simulink model "P702_NI_SoftECU"  (R2019a)
settings: Solver=ode1  StartTime=0.0  StopTime=Inf  FixedStep=0.001  RelTol=1e-3  EnableMultiTasking=on
PreLoadFcn:
  | run '.\VeriStand_BlockSet\NIVeriStandAddPaths.m'
undefined symbols (not defined in the file or in its folder): magnitude
libraries: simulink x83, simulink_extras x1
(part 64 of 76)

== system P702_NI_SoftECU/Output/Subsystem1/CAN_Signal/ABS_ESC/Global_PATS_SubTarget_0x49 ==
  in_port : Inport
  bus_selector : BusSelector  OutputSignals=immoSubTarget1Cmd_T1,immoSubTarget1Data_T1
  immoSubTarget1Cmd_T1 : Terminator
  immoSubTarget1Data_T1 : Terminator
  wires:
  in_port/1 -> bus_selector/1  "Subsystem1"
  bus_selector/1 -> immoSubTarget1Cmd_T1/1  "<immoSubTarget1Cmd_T1>"
  bus_selector/2 -> immoSubTarget1Data_T1/1  "<immoSubTarget1Data_T1>"

== system P702_NI_SoftECU/Output/Subsystem1/CAN_Signal/ABS_ESC/SelectDriveModeData2_0x44E ==
  in_port : Inport
  SelDrvMdePos01_D_Stat : Terminator
  SelDrvMdePos02_D_Stat : Terminator
  SelDrvMdePos03_D_Stat : Terminator
  SelDrvMdePos04_D_Stat : Terminator
  SelDrvMdePos05_D_Stat : Terminator
  SelDrvMdePos06_D_Stat : Terminator
  SelDrvMdePos07_D_Stat : Terminator
  SelDrvMdePos08_D_Stat : Terminator
  SelDrvMdePos09_D_Stat : Terminator
  SelDrvMdePos10_D_Stat : Terminator
  SelDrvMdePos11_D_Stat : Terminator
  SelDrvMdePos12_D_Stat : Terminator
  bus_selector : BusSelector  OutputSignals=SelDrvMdePos01_D_Stat,SelDrvMdePos02_D_Stat,SelDrvMdePos03_D_Stat,SelDrvMdePos04_D_Stat,SelDrvMdePos05_D_Stat,SelDrvMdePos06_D_Stat,SelDrvMdePos07_D_Stat,SelDrvMdePos12_D_Stat,SelDrvMdePos11_D_Stat,SelDrvMdePos10_D_Stat,SelDrvMdePos09_D_Stat,SelDrvMdePos08_D_Stat
  wires:
  in_port/1 -> bus_selector/1  "Subsystem1"
  bus_selector/1 -> SelDrvMdePos01_D_Stat/1  "<SelDrvMdePos01_D_Stat>"
  bus_selector/2 -> SelDrvMdePos02_D_Stat/1  "<SelDrvMdePos02_D_Stat>"
  bus_selector/3 -> SelDrvMdePos03_D_Stat/1  "<SelDrvMdePos03_D_Stat>"
  bus_selector/4 -> SelDrvMdePos04_D_Stat/1  "<SelDrvMdePos04_D_Stat>"
  bus_selector/5 -> SelDrvMdePos05_D_Stat/1  "<SelDrvMdePos05_D_Stat>"
  bus_selector/6 -> SelDrvMdePos06_D_Stat/1  "<SelDrvMdePos06_D_Stat>"
  bus_selector/7 -> SelDrvMdePos07_D_Stat/1  "<SelDrvMdePos07_D_Stat>"
  bus_selector/8 -> SelDrvMdePos12_D_Stat/1  "<SelDrvMdePos12_D_Stat>"
  bus_selector/9 -> SelDrvMdePos11_D_Stat/1  "<SelDrvMdePos11_D_Stat>"
  bus_selector/10 -> SelDrvMdePos10_D_Stat/1  "<SelDrvMdePos10_D_Stat>"
  bus_selector/11 -> SelDrvMdePos09_D_Stat/1  "<SelDrvMdePos09_D_Stat>"
  bus_selector/12 -> SelDrvMdePos08_D_Stat/1  "<SelDrvMdePos08_D_Stat>"

== system P702_NI_SoftECU/Output/Subsystem1/CAN_Signal/ABS_ESC/SelectDriveModeData_0x420 ==
  in_port : Inport
  ActvDrvMde_D2_Stat : Terminator
  AwdMde_D_RqBrk : Terminator
  SelDrvMdeMsgTxt_D_Rq : Terminator
  SelDrvMdePos01_B_Avail : Terminator
  SelDrvMdePos02_B_Avail : Terminator
  SelDrvMdePos03_B_Avail : Terminator
  SelDrvMdePos04_B_Avail : Terminator
  SelDrvMdePos05_B_Avail : Terminator
  SelDrvMdePos06_B_Avail : Terminator
  SelDrvMdePos07_B_Avail : Terminator
  SelDrvMdePos08_B_Avail : Terminator
  SelDrvMdePos09_B_Avail : Terminator
  SelDrvMdePos10_B_Avail : Terminator
  SelDrvMdePos11_B_Avail : Terminator
  SelDrvMdePos12_B_Avail : Terminator
  SelDrvMdePt_D_Rq : Terminator
  SelDrvMde_D2_Rq : Terminator
  SelDrvMde_D_Stat : Terminator
  bus_selector : BusSelector  OutputSignals=SelDrvMdeMsgTxt_D_Rq,SelDrvMdePt_D_Rq,SelDrvMde_D_Stat,SelDrvMdePos01_B_Avail,AwdMde_D_RqBrk,SelDrvMdePos02_B_Avail,SelDrvMdePos03_B_Avail,SelDrvMdePos04_B_Avail,SelDrvMdePos05_B_Avail,SelDrvMdePos06_B_Avail,SelDrvMdePos07_B_Avail,SelDrvMdePos08_B_Avail,SelDrvMdePos09_B_Avail,SelDrvMdePos10_B_Avail,SelDrvMdePos11_B_Avail,SelDrvMdePos12_B_Avail,ActvDrvMde_D2_Stat,SelDrvMde_D2_Rq
  wires:
  in_port/1 -> bus_selector/1  "Subsystem1"
  bus_selector/1 -> SelDrvMdeMsgTxt_D_Rq/1  "<SelDrvMdeMsgTxt_D_Rq>"
  bus_selector/2 -> SelDrvMdePt_D_Rq/1  "<SelDrvMdePt_D_Rq>"
  bus_selector/3 -> SelDrvMde_D_Stat/1  "<SelDrvMde_D_Stat>"
  bus_selector/4 -> SelDrvMdePos01_B_Avail/1  "<SelDrvMdePos01_B_Avail>"
  bus_selector/5 -> AwdMde_D_RqBrk/1  "<AwdMde_D_RqBrk>"
  bus_selector/6 -> SelDrvMdePos02_B_Avail/1  "<SelDrvMdePos02_B_Avail>"
  bus_selector/7 -> SelDrvMdePos03_B_Avail/1  "<SelDrvMdePos03_B_Avail>"
  bus_selector/8 -> SelDrvMdePos04_B_Avail/1  "<SelDrvMdePos04_B_Avail>"
  bus_selector/9 -> SelDrvMdePos05_B_Avail/1  "<SelDrvMdePos05_B_Avail>"
  bus_selector/10 -> SelDrvMdePos06_B_Avail/1  "<SelDrvMdePos06_B_Avail>"
  bus_selector/11 -> SelDrvMdePos07_B_Avail/1  "<SelDrvMdePos07_B_Avail>"
  bus_selector/12 -> SelDrvMdePos08_B_Avail/1  "<SelDrvMdePos08_B_Avail>"
  bus_selector/13 -> SelDrvMdePos09_B_Avail/1  "<SelDrvMdePos09_B_Avail>"
  bus_selector/14 -> SelDrvMdePos10_B_Avail/1  "<SelDrvMdePos10_B_Avail>"
  bus_selector/15 -> SelDrvMdePos11_B_Avail/1  "<SelDrvMdePos11_B_Avail>"
  bus_selector/16 -> SelDrvMdePos12_B_Avail/1  "<SelDrvMdePos12_B_Avail>"
  bus_selector/17 -> ActvDrvMde_D2_Stat/1  "<ActvDrvMde_D2_Stat>"
  bus_selector/18 -> SelDrvMde_D2_Rq/1  "<SelDrvMde_D2_Rq>"

== system P702_NI_SoftECU/Output/Subsystem1/CAN_Signal/ABS_ESC/SteeringPinion_Data2_0x7F ==
  in_port : Inport
  AwdLatDelta_B_Rq : Terminator
  AwdLatDelta_Tq_Rq : Terminator
  bus_selector : BusSelector  OutputSignals=AwdLatDelta_B_Rq,AwdLatDelta_Tq_Rq
  wires:
  in_port/1 -> bus_selector/1  "Subsystem1"
  bus_selector/1 -> AwdLatDelta_B_Rq/1  "<AwdLatDelta_B_Rq>"
  bus_selector/2 -> AwdLatDelta_Tq_Rq/1  "<AwdLatDelta_Tq_Rq>"

== system P702_NI_SoftECU/Output/Subsystem1/CAN_Signal/ABS_ESC/TesterPhysicalResABS_0x768 ==
  in_port : Inport
  TesterPhysicalResABS : Terminator
  bus_selector : BusSelector  OutputSignals=TesterPhysicalResABS
  wires:
  in_port/1 -> bus_selector/1  "Subsystem1"
  bus_selector/1 -> TesterPhysicalResABS/1  "<TesterPhysicalResABS>"

== system P702_NI_SoftECU/Output/Subsystem1/CAN_Signal/ABS_ESC/TrailerBrakeData_0x412 ==
  in_port : Inport
  TrlrBrk_Pc_Rq : Terminator
  VehPtch_An_Dsply : Terminator
  VehRol_An_Dsply : Terminator
  bus_selector : BusSelector  OutputSignals=TrlrBrk_Pc_Rq,VehPtch_An_Dsply,VehRol_An_Dsply
  wires:
  in_port/1 -> bus_selector/1  "Subsystem1"
  bus_selector/1 -> TrlrBrk_Pc_Rq/1  "<TrlrBrk_Pc_Rq>"
  bus_selector/2 -> VehPtch_An_Dsply/1  "<VehPtch_An_Dsply>"
  bus_selector/3 -> VehRol_An_Dsply/1  "<VehRol_An_Dsply>"

== system P702_NI_SoftECU/Output/Subsystem1/CAN_Signal/ABS_ESC/WheelData_0x216 ==
  in_port : Inport
  BrkObdData_No_Actl : Terminator
  BrkObdIndex_No_Actl : Terminator
  WhlDirFl_D_Actl : Terminator
  WhlDirFr_D_Actl : Terminator
  WhlDirRl_D_Actl : Terminator
  WhlDirRr_D_Actl : Terminator
  WhlRotatFl_No_Cnt : Terminator
  WhlRotatFr_No_Cnt : Terminator
  WhlRotatRl_No_Cnt : Terminator
  WhlRotatRr_No_Cnt : Terminator
  bus_selector : BusSelector  OutputSignals=WhlRotatFr_No_Cnt,WhlRotatFl_No_Cnt,WhlRotatRr_No_Cnt,WhlRotatRl_No_Cnt,WhlDirRl_D_Actl,WhlDirFr_D_Actl,WhlDirFl_D_Actl,WhlDirRr_D_Actl,BrkObdIndex_No_Actl,BrkObdData_No_Actl
  wires:
  in_port/1 -> bus_selector/1  "Subsystem1"
  bus_selector/1 -> WhlRotatFr_No_Cnt/1  "<WhlRotatFr_No_Cnt>"
  bus_selector/2 -> WhlRotatFl_No_Cnt/1  "<WhlRotatFl_No_Cnt>"
  bus_selector/3 -> WhlRotatRr_No_Cnt/1  "<WhlRotatRr_No_Cnt>"
  bus_selector/4 -> WhlRotatRl_No_Cnt/1  "<WhlRotatRl_No_Cnt>"
  bus_selector/5 -> WhlDirRl_D_Actl/1  "<WhlDirRl_D_Actl>"
  bus_selector/6 -> WhlDirFr_D_Actl/1  "<WhlDirFr_D_Actl>"
  bus_selector/7 -> WhlDirFl_D_Actl/1  "<WhlDirFl_D_Actl>"
  bus_selector/8 -> WhlDirRr_D_Actl/1  "<WhlDirRr_D_Actl>"
  bus_selector/9 -> BrkObdIndex_No_Actl/1  "<BrkObdIndex_No_Actl>"
  bus_selector/10 -> BrkObdData_No_Actl/1  "<BrkObdData_No_Actl>"

== system P702_NI_SoftECU/Output/Subsystem1/CAN_Signal/ABS_ESC/WheelSpeed_0x217 ==
  in_port : Inport
  WhlFl_W_Meas : Terminator
  WhlFr_W_Meas : Terminator
  WhlRl_W_Meas : Terminator
  WhlRr_W_Meas : Terminator
  bus_selector : BusSelector  OutputSignals=WhlFl_W_Meas,WhlFr_W_Meas,WhlRl_W_Meas,WhlRr_W_Meas
  wires:
  in_port/1 -> bus_selector/1  "Subsystem1"
  bus_selector/1 -> WhlFl_W_Meas/1  "<WhlFl_W_Meas>"
  bus_selector/2 -> WhlFr_W_Meas/1  "<WhlFr_W_Meas>"
  bus_selector/3 -> WhlRl_W_Meas/1  "<WhlRl_W_Meas>"
  bus_selector/4 -> WhlRr_W_Meas/1  "<WhlRr_W_Meas>"

== system P702_NI_SoftECU/Output/Subsystem1/CAN_Signal/ADAS/ACCDATA ==
  in_port : Inport
  AccBrkDecel_B_Rq : Terminator
  AccBrkPrchg_B_Rq : Terminator
  AccBrkTot_A_Rq : Terminator
  AccCancl_B_Rq : Terminator
  AccPrpl_A_Rq : Terminator
  AccPrpl_A_Rq1 : Terminator
  AccStopStat_B_Rq : Terminator
  CmbbEngTqMn_B_Rq : Terminator
  bus_selector : BusSelector  OutputSignals=AccBrkPrchg_B_Rq,AccBrkDecel_B_Rq,AccStopStat_B_Rq,AccBrkTot_A_Rq,CmbbEngTqMn_B_Rq,AccCancl_B_Rq,AccPrpl_A_Rq,AccPrpl_A_Rq1
  wires:
  in_port/1 -> bus_selector/1  "Subsystem1"
  bus_selector/1 -> AccBrkPrchg_B_Rq/1  "<AccBrkPrchg_B_Rq>"
  bus_selector/2 -> AccBrkDecel_B_Rq/1  "<AccBrkDecel_B_Rq>"
  bus_selector/3 -> AccStopStat_B_Rq/1  "<AccStopStat_B_Rq>"
  bus_selector/4 -> AccBrkTot_A_Rq/1  "<AccBrkTot_A_Rq>"
  bus_selector/5 -> CmbbEngTqMn_B_Rq/1  "<CmbbEngTqMn_B_Rq>"
  bus_selector/6 -> AccCancl_B_Rq/1  "<AccCancl_B_Rq>"
  bus_selector/7 -> AccPrpl_A_Rq/1  "<AccPrpl_A_Rq>"
  bus_selector/8 -> AccPrpl_A_Rq1/1  "<AccPrpl_A_Rq1>"

== system P702_NI_SoftECU/Output/Subsystem1/CAN_Signal/ADAS/ACCDATA_2 ==
  in_port : Inport
  CmbbBaSens_D_Rq : Terminator
  CmbbBrkDecel_A_Rq : Terminator
  CmbbBrkDecel_B_Rq : Terminator
  CmbbBrkPrchg_D_Rq : Terminator
  bus_selector : BusSelector  OutputSignals=CmbbBrkPrchg_D_Rq,CmbbBrkDecel_A_Rq,CmbbBaSens_D_Rq,CmbbBrkDecel_B_Rq
  wires:
  in_port/1 -> bus_selector/1  "Subsystem1"
  bus_selector/1 -> CmbbBrkPrchg_D_Rq/1  "<CmbbBrkPrchg_D_Rq>"
  bus_selector/2 -> CmbbBrkDecel_A_Rq/1  "<CmbbBrkDecel_A_Rq>"
  bus_selector/3 -> CmbbBaSens_D_Rq/1  "<CmbbBaSens_D_Rq>"
  bus_selector/4 -> CmbbBrkDecel_B_Rq/1  "<CmbbBrkDecel_B_Rq>"

== system P702_NI_SoftECU/Output/Subsystem1/CAN_Signal/BCM/BCM_Lamp_Stat_0x3C3 ==
  in_port : Inport
  BrkWarnInd_B_Rq : Terminator
  Brk_Fluid_Lvl_Low : Terminator
  Courtesy_BSave_Stat : Terminator
  Courtesy_Delay_Status : Terminator
  CrnrLghtLeft_Pc_Rq : Terminator
  CrnrLghtRight_Pc_Rq : Terminator
  DayRnngLampOn_B_Stat : Terminator
  DrTgateLck_D_Stat : Terminator
  Dr_Courtesy_Light_Stat : Terminator
  HeadLampLoActv_B_Stat : Terminator
  HeadLampLoFlOn_B_Stat : Terminator
  HeadLampLoFrOn_B_Stat : Terminator
  HeadLampLoOut_B_Stat : Terminator
  HeadLghtHiFdbck_D_Stat : Terminator
  HeadLghtHiOn_B_Stat : Terminator
  HeadLghtSwtch_D_Stat : Terminator
  Headlamp_On_Wrning_Cmd : Terminator
  HomeSafeLtChime_B_Rq : Terminator
  Illuminated_Entry_Stat : Terminator
  ImpactEvntFdbck_D_Stat : Terminator
  KeyInIgnWarn_B_Cmd : Terminator
  Park_Brake_Chime_Rqst : Terminator
  PerimeterAlarmChimeRq : Terminator
  Perimeter_Alarm_Status : Terminator
  PrkLght_D_Stat : Terminator
  PrkLightChime_B_Rq : Terminator
  PudLampDrv_D_Rq : Terminator
  PudLampPsngr_D_Rq : Terminator
  PudLamp_D_Rq : Terminator
  ReducedGuard_D_Stat : Terminator
  RvrseLghtOn_B_Stat : Terminator
  StopLghtOn_B_Stat : Terminator
  TrnNotInPrkChime_B_Rq : Terminator
  WndwGlbl_D_Cmd : Terminator
  WrlssAcsyChrgInhbt_B_Rq : Terminator
  bus_selector : BusSelector  OutputSignals=BrkWarnInd_B_Rq,Brk_Fluid_Lvl_Low,Courtesy_BSave_Stat,Courtesy_Delay_Status,CrnrLghtLeft_Pc_Rq,CrnrLghtRight_Pc_Rq,DayRnngLampOn_B_Stat,DrTgateLck_D_Stat,Dr_Courtesy_Light_Stat,HeadLampLoActv_B_Stat,HeadLampLoFlOn_B_Stat,HeadLampLoFrOn_B_Stat,HeadLampLoOut_B_Stat,HeadLghtHiFdbck_D_Stat,HeadLghtHiOn_B_Stat,HeadLghtSwtch_D_Stat,Headlamp_On_Wrning_Cmd,HomeSafeLtChime_B_Rq,Illuminated_Entry_Stat,ImpactEvntFdbck_D_Stat,KeyInIgnWarn_B_Cmd,Park_Brake_Chime_Rqst,PerimeterAlarmChimeRq,Perimeter_Alarm_Status,PrkLght_D_Stat,PrkLightChime_B_Rq,PudLampDrv_D_Rq,PudLampPsngr_D_Rq,PudLamp_D_Rq,ReducedGuard_D_Stat,RvrseLghtOn_B_Stat,StopLghtOn_B_Stat,TrnNotInPrkChime_B_Rq,WndwGlbl_D_Cmd,WrlssAcsyChrgInhbt_B_Rq
  wires:
  in_port/1 -> bus_selector/1  "Subsystem1"
  bus_selector/1 -> BrkWarnInd_B_Rq/1  "<BrkWarnInd_B_Rq>"
  bus_selector/2 -> Brk_Fluid_Lvl_Low/1  "<Brk_Fluid_Lvl_Low>"
  bus_selector/3 -> Courtesy_BSave_Stat/1  "<Courtesy_BSave_Stat>"
  bus_selector/4 -> Courtesy_Delay_Status/1  "<Courtesy_Delay_Status>"
  bus_selector/5 -> CrnrLghtLeft_Pc_Rq/1  "<CrnrLghtLeft_Pc_Rq>"
  bus_selector/6 -> CrnrLghtRight_Pc_Rq/1  "<CrnrLghtRight_Pc_Rq>"
  bus_selector/7 -> DayRnngLampOn_B_Stat/1  "<DayRnngLampOn_B_Stat>"
  bus_selector/8 -> DrTgateLck_D_Stat/1  "<DrTgateLck_D_Stat>"
  bus_selector/9 -> Dr_Courtesy_Light_Stat/1  "<Dr_Courtesy_Light_Stat>"
  bus_selector/10 -> HeadLampLoActv_B_Stat/1  "<HeadLampLoActv_B_Stat>"
  bus_selector/11 -> HeadLampLoFlOn_B_Stat/1  "<HeadLampLoFlOn_B_Stat>"
  bus_selector/12 -> HeadLampLoFrOn_B_Stat/1  "<HeadLampLoFrOn_B_Stat>"
  bus_selector/13 -> HeadLampLoOut_B_Stat/1  "<HeadLampLoOut_B_Stat>"
  bus_selector/14 -> HeadLghtHiFdbck_D_Stat/1  "<HeadLghtHiFdbck_D_Stat>"
  bus_selector/15 -> HeadLghtHiOn_B_Stat/1  "<HeadLghtHiOn_B_Stat>"
  bus_selector/16 -> HeadLghtSwtch_D_Stat/1  "<HeadLghtSwtch_D_Stat>"
  bus_selector/17 -> Headlamp_On_Wrning_Cmd/1  "<Headlamp_On_Wrning_Cmd>"
  bus_selector/18 -> HomeSafeLtChime_B_Rq/1  "<HomeSafeLtChime_B_Rq>"
  bus_selector/19 -> Illuminated_Entry_Stat/1  "<Illuminated_Entry_Stat>"
  bus_selector/20 -> ImpactEvntFdbck_D_Stat/1  "<ImpactEvntFdbck_D_Stat>"
  bus_selector/21 -> KeyInIgnWarn_B_Cmd/1  "<KeyInIgnWarn_B_Cmd>"
  bus_selector/22 -> Park_Brake_Chime_Rqst/1  "<Park_Brake_Chime_Rqst>"
  bus_selector/23 -> PerimeterAlarmChimeRq/1  "<PerimeterAlarmChimeRq>"
  bus_selector/24 -> Perimeter_Alarm_Status/1  "<Perimeter_Alarm_Status>"
  bus_selector/25 -> PrkLght_D_Stat/1  "<PrkLght_D_Stat>"
  bus_selector/26 -> PrkLightChime_B_Rq/1  "<PrkLightChime_B_Rq>"
  bus_selector/27 -> PudLampDrv_D_Rq/1  "<PudLampDrv_D_Rq>"
  bus_selector/28 -> PudLampPsngr_D_Rq/1  "<PudLampPsngr_D_Rq>"
  bus_selector/29 -> PudLamp_D_Rq/1  "<PudLamp_D_Rq>"
  bus_selector/30 -> ReducedGuard_D_Stat/1  "<ReducedGuard_D_Stat>"
  bus_selector/31 -> RvrseLghtOn_B_Stat/1  "<RvrseLghtOn_B_Stat>"
  bus_selector/32 -> StopLghtOn_B_Stat/1  "<StopLghtOn_B_Stat>"
  bus_selector/33 -> TrnNotInPrkChime_B_Rq/1  "<TrnNotInPrkChime_B_Rq>"
  bus_selector/34 -> WndwGlbl_D_Cmd/1  "<WndwGlbl_D_Cmd>"
  bus_selector/35 -> WrlssAcsyChrgInhbt_B_Rq/1  "<WrlssAcsyChrgInhbt_B_Rq>"

== system P702_NI_SoftECU/Output/Subsystem1/CAN_Signal/BCM/Battery_Mgmt_24V_0x42E ==
  in_port : Inport
  BattULo24Soc_Pc_Actl : Terminator
  BattULo24State_D_Qlty : Terminator
  BattULo24_Ah_DeltaRide : Terminator
  BattULo24_B_Falt : Terminator
  BattULo24_I_Actl : Terminator
  bus_selector : BusSelector  OutputSignals=BattULo24_Ah_DeltaRide,BattULo24_B_Falt,BattULo24_I_Actl,BattULo24State_D_Qlty,BattULo24Soc_Pc_Actl
  wires:
  in_port/1 -> bus_selector/1  "Subsystem1"
  bus_selector/1 -> BattULo24_Ah_DeltaRide/1  "<BattULo24_Ah_DeltaRide>"
  bus_selector/2 -> BattULo24_B_Falt/1  "<BattULo24_B_Falt>"
  bus_selector/3 -> BattULo24_I_Actl/1  "<BattULo24_I_Actl>"
  bus_selector/4 -> BattULo24State_D_Qlty/1  "<BattULo24State_D_Qlty>"
  bus_selector/5 -> BattULo24Soc_Pc_Actl/1  "<BattULo24Soc_Pc_Actl>"

== system P702_NI_SoftECU/Output/Subsystem1/CAN_Signal/BCM/Battery_Mgmt_2_0x42C ==
  in_port : Inport
  BattULoChrg_D_Rq : Terminator
  BattULoSrvc_T_Actl : Terminator
  Batt_Crit_SoC_B : Terminator
  Batt_Lo_SoC_B : Terminator
  ChargeMode : Terminator
  EngStrtInhbt_B_RqBatt : Terminator
  IdleSpeedIncrease_El : Terminator
  PeriodicElLoad_B_Stat : Terminator
  PwSysULoFalt_D_Stat : Terminator
  Shed_Drain_Eng_Off_B : Terminator
  Shed_Feature_Group_ID : Terminator
  Shed_Level_Req : Terminator
  Shed_T_Eng_Off_B : Terminator
  ULoRgenTestMde_B_Rq : Terminator
  bus_selector : BusSelector  OutputSignals=BattULoChrg_D_Rq,BattULoSrvc_T_Actl,Batt_Crit_SoC_B,Batt_Lo_SoC_B,ChargeMode,EngStrtInhbt_B_RqBatt,IdleSpeedIncrease_El,PeriodicElLoad_B_Stat,PwSysULoFalt_D_Stat,Shed_Drain_Eng_Off_B,Shed_Feature_Group_ID,Shed_Level_Req,Shed_T_Eng_Off_B,ULoRgenTestMde_B_Rq
  wires:
  in_port/1 -> bus_selector/1  "Subsystem1"
  bus_selector/1 -> BattULoChrg_D_Rq/1  "<BattULoChrg_D_Rq>"
  bus_selector/2 -> BattULoSrvc_T_Actl/1  "<BattULoSrvc_T_Actl>"
  bus_selector/3 -> Batt_Crit_SoC_B/1  "<Batt_Crit_SoC_B>"
  bus_selector/4 -> Batt_Lo_SoC_B/1  "<Batt_Lo_SoC_B>"
  bus_selector/5 -> ChargeMode/1  "<ChargeMode>"
  bus_selector/6 -> EngStrtInhbt_B_RqBatt/1  "<EngStrtInhbt_B_RqBatt>"
  bus_selector/7 -> IdleSpeedIncrease_El/1  "<IdleSpeedIncrease_El>"
  bus_selector/8 -> PeriodicElLoad_B_Stat/1  "<PeriodicElLoad_B_Stat>"
  bus_selector/9 -> PwSysULoFalt_D_Stat/1  "<PwSysULoFalt_D_Stat>"
  bus_selector/10 -> Shed_Drain_Eng_Off_B/1  "<Shed_Drain_Eng_Off_B>"
  bus_selector/11 -> Shed_Feature_Group_ID/1  "<Shed_Feature_Group_ID>"
  bus_selector/12 -> Shed_Level_Req/1  "<Shed_Level_Req>"
  bus_selector/13 -> Shed_T_Eng_Off_B/1  "<Shed_T_Eng_Off_B>"
  bus_selector/14 -> ULoRgenTestMde_B_Rq/1  "<ULoRgenTestMde_B_Rq>"

== system P702_NI_SoftECU/Output/Subsystem1/CAN_Signal/BCM/Battery_Mgmt_3_0x43C ==
  in_port : Inport
  BSBattQCapAh : Terminator
  BSBattQDeltaRideAh : Terminator
  BSBattSOC : Terminator
  BSFault : Terminator
  BattULo2_Te_Actl : Terminator
  BattULoChrg_URate_RqMx : Terminator
  BattULoChrg_U_RqMn : Terminator
  BattULoChrg_U_RqMx : Terminator
  BattULoState_D_Qlty : Terminator
  bus_selector : BusSelector  OutputSignals=BSFault,BSBattQDeltaRideAh,BSBattSOC,BattULo2_Te_Actl,BSBattQCapAh,BattULoState_D_Qlty,BattULoChrg_U_RqMn,BattULoChrg_U_RqMx,BattULoChrg_URate_RqMx
  wires:
  in_port/1 -> bus_selector/1  "Subsystem1"
  bus_selector/1 -> BSFault/1  "<BSFault>"
  bus_selector/2 -> BSBattQDeltaRideAh/1  "<BSBattQDeltaRideAh>"
  bus_selector/3 -> BSBattSOC/1  "<BSBattSOC>"
  bus_selector/4 -> BattULo2_Te_Actl/1  "<BattULo2_Te_Actl>"
  bus_selector/5 -> BSBattQCapAh/1  "<BSBattQCapAh>"
  bus_selector/6 -> BattULoState_D_Qlty/1  "<BattULoState_D_Qlty>"
  bus_selector/7 -> BattULoChrg_U_RqMn/1  "<BattULoChrg_U_RqMn>"
  bus_selector/8 -> BattULoChrg_U_RqMx/1  "<BattULoChrg_U_RqMx>"
  bus_selector/9 -> BattULoChrg_URate_RqMx/1  "<BattULoChrg_URate_RqMx>"

== system P702_NI_SoftECU/Output/Subsystem1/CAN_Signal/BCM/Battery_Mgmt_4_0x42B ==
  in_port : Inport
  BattULoAuxSoc_Pc_Actl : Terminator
  BattULoAux_B_Falt : Terminator
  BattULoAux_D_Qlty : Terminator
  BattULoAux_I_Actl : Terminator
  BattULoAux_U_Actl : Terminator
  BattULoCrnkBelt_U_Pred : Terminator
  BattULoCrnkStrt_U_Pred : Terminator
  bus_selector : BusSelector  OutputSignals=BattULoAux_U_Actl,BattULoAuxSoc_Pc_Actl,BattULoAux_B_Falt,BattULoAux_I_Actl,BattULoAux_D_Qlty,BattULoCrnkBelt_U_Pred,BattULoCrnkStrt_U_Pred
  wires:
  in_port/1 -> bus_selector/1  "Subsystem1"
  bus_selector/1 -> BattULoAux_U_Actl/1  "<BattULoAux_U_Actl>"
  bus_selector/2 -> BattULoAuxSoc_Pc_Actl/1  "<BattULoAuxSoc_Pc_Actl>"
  bus_selector/3 -> BattULoAux_B_Falt/1  "<BattULoAux_B_Falt>"
  bus_selector/4 -> BattULoAux_I_Actl/1  "<BattULoAux_I_Actl>"
  bus_selector/5 -> BattULoAux_D_Qlty/1  "<BattULoAux_D_Qlty>"
  bus_selector/6 -> BattULoCrnkBelt_U_Pred/1  "<BattULoCrnkBelt_U_Pred>"
  bus_selector/7 -> BattULoCrnkStrt_U_Pred/1  "<BattULoCrnkStrt_U_Pred>"

== system P702_NI_SoftECU/Output/Subsystem1/CAN_Signal/BCM/BodyInfo_3_0x3B3 ==
  in_port : Inport
  Backlit_LED_Status : Terminator
  BodySrvcRqd_B_Rq : Terminator
  CrashEvnt_D_Stat : Terminator
  Day_Night_Status : Terminator
  Delay_Accy : Terminator
  DimmingLvlEvnt_No_Actl : Terminator
  Dimming_Lvl : Terminator
  DrStatDrvErrCnt_B_Stat : Terminator
  DrStatDrv_B_Actl : Terminator
  DrStatHood_B_Actl : Terminator
  DrStatInnrTgate_B_Actl : Terminator
  DrStatPsngr_B_Actl : Terminator
  DrStatRl_B_Actl : Terminator
  DrStatRr_B_Actl : Terminator
  DrStatTgate_B_Actl : Terminator
  FogLghtFrontOn_B_Stat : Terminator
  FogLghtRearOn_B_Stat : Terminator
  FuelPmpInhbt_B_Stat : Terminator
  IgnKeyType_D_Actl : Terminator
  Ignition_Status : Terminator
  Key_In_Ignition_Stat : Terminator
  LifeCycMde_D_Actl : Terminator
  Litval : Terminator
  Parklamp_Status : Terminator
  PrkBrkActv_B_Actl : Terminator
  Remote_Start_Status : Terminator
  TurnLghtLeftOn_B_Stat : Terminator
  TurnLghtLeft_D_Rq : Terminator
  TurnLghtRightOn_B_Stat : Terminator
  TurnLghtRight_D_Rq : Terminator
  ValetMode_D_Mem : Terminator
  bus_selector : BusSelector  OutputSignals=Ignition_Status,Parklamp_Status,FogLghtRearOn_B_Stat,DrStatTgate_B_Actl,Day_Night_Status,Remote_Start_Status,Key_In_Ignition_Stat,BodySrvcRqd_B_Rq,TurnLghtLeft_D_Rq,Backlit_LED_Status,DrStatDrvErrCnt_B_Stat,DimmingLvlEvnt_No_Actl,ValetMode_D_Mem,Dimming_Lvl,IgnKeyType_D_Actl,TurnLghtRightOn_B_Stat,CrashEvnt_D_Stat,FuelPmpInhbt_B_Stat,Litval,PrkBrkActv_B_Actl,TurnLghtLeftOn_B_Stat,LifeCycMde_D_Actl,DrStatRr_B_Actl,DrStatRl_B_Actl,TurnLghtRight_D_Rq,DrStatDrv_B_Actl,DrStatPsngr_B_Actl,DrStatHood_B_Actl,DrStatInnrTgate_B_Actl,Delay_Accy,FogLghtFrontOn_B_Stat
  wires:
  in_port/1 -> bus_selector/1  "Subsystem1"
  bus_selector/1 -> Ignition_Status/1  "<Ignition_Status>"
  bus_selector/2 -> Parklamp_Status/1  "<Parklamp_Status>"
  bus_selector/3 -> FogLghtRearOn_B_Stat/1  "<FogLghtRearOn_B_Stat>"
  bus_selector/4 -> DrStatTgate_B_Actl/1  "<DrStatTgate_B_Actl>"
  bus_selector/5 -> Day_Night_Status/1  "<Day_Night_Status>"
  bus_selector/6 -> Remote_Start_Status/1  "<Remote_Start_Status>"
  bus_selector/7 -> Key_In_Ignition_Stat/1  "<Key_In_Ignition_Stat>"
  bus_selector/8 -> BodySrvcRqd_B_Rq/1  "<BodySrvcRqd_B_Rq>"
  bus_selector/9 -> TurnLghtLeft_D_Rq/1  "<TurnLghtLeft_D_Rq>"
  bus_selector/10 -> Backlit_LED_Status/1  "<Backlit_LED_Status>"
  bus_selector/11 -> DrStatDrvErrCnt_B_Stat/1  "<DrStatDrvErrCnt_B_Stat>"
  bus_selector/12 -> DimmingLvlEvnt_No_Actl/1  "<DimmingLvlEvnt_No_Actl>"
  bus_selector/13 -> ValetMode_D_Mem/1  "<ValetMode_D_Mem>"
  bus_selector/14 -> Dimming_Lvl/1  "<Dimming_Lvl>"
  bus_selector/15 -> IgnKeyType_D_Actl/1  "<IgnKeyType_D_Actl>"
  bus_selector/16 -> TurnLghtRightOn_B_Stat/1  "<TurnLghtRightOn_B_Stat>"
  bus_selector/17 -> CrashEvnt_D_Stat/1  "<CrashEvnt_D_Stat>"
  bus_selector/18 -> FuelPmpInhbt_B_Stat/1  "<FuelPmpInhbt_B_Stat>"
  bus_selector/19 -> Litval/1  "<Litval>"
  bus_selector/20 -> PrkBrkActv_B_Actl/1  "<PrkBrkActv_B_Actl>"
  bus_selector/21 -> TurnLghtLeftOn_B_Stat/1  "<TurnLghtLeftOn_B_Stat>"
  bus_selector/22 -> LifeCycMde_D_Actl/1  "<LifeCycMde_D_Actl>"
  bus_selector/23 -> DrStatRr_B_Actl/1  "<DrStatRr_B_Actl>"
  bus_selector/24 -> DrStatRl_B_Actl/1  "<DrStatRl_B_Actl>"
  bus_selector/25 -> TurnLghtRight_D_Rq/1  "<TurnLghtRight_D_Rq>"
  bus_selector/26 -> DrStatDrv_B_Actl/1  "<DrStatDrv_B_Actl>"
  bus_selector/27 -> DrStatPsngr_B_Actl/1  "<DrStatPsngr_B_Actl>"
  bus_selector/28 -> DrStatHood_B_Actl/1  "<DrStatHood_B_Actl>"
  bus_selector/29 -> DrStatInnrTgate_B_Actl/1  "<DrStatInnrTgate_B_Actl>"
  bus_selector/30 -> Delay_Accy/1  "<Delay_Accy>"
  bus_selector/31 -> FogLghtFrontOn_B_Stat/1  "<FogLghtFrontOn_B_Stat>"

== system P702_NI_SoftECU/Output/Subsystem1/CAN_Signal/BCM/Body_Info_10_0x3BA ==
  in_port : Inport
  GenericSwtch1_No_Actl : Terminator
  GenericSwtch2_No_Actl : Terminator
  GenericSwtch3_No_Actl : Terminator
  bus_selector : BusSelector  OutputSignals=GenericSwtch1_No_Actl,GenericSwtch2_No_Actl,GenericSwtch3_No_Actl
  wires:
  in_port/1 -> bus_selector/1  "Subsystem1"
  bus_selector/1 -> GenericSwtch1_No_Actl/1  "<GenericSwtch1_No_Actl>"
  bus_selector/2 -> GenericSwtch2_No_Actl/1  "<GenericSwtch2_No_Actl>"
  bus_selector/3 -> GenericSwtch3_No_Actl/1  "<GenericSwtch3_No_Actl>"

== system P702_NI_SoftECU/Output/Subsystem1/CAN_Signal/BCM/Body_Info_12_0x26E ==
  in_port : Inport
  FobCtlPssvData_No_Actl : Terminator
  FobCtlRollCode_No_Stat : Terminator
  FobCtlType_D_Stat : Terminator
  bus_selector : BusSelector  OutputSignals=FobCtlPssvData_No_Actl,FobCtlRollCode_No_Stat,FobCtlType_D_Stat
  wires:
  in_port/1 -> bus_selector/1  "Subsystem1"
  bus_selector/1 -> FobCtlPssvData_No_Actl/1  "<FobCtlPssvData_No_Actl>"
  bus_selector/2 -> FobCtlRollCode_No_Stat/1  "<FobCtlRollCode_No_Stat>"
  bus_selector/3 -> FobCtlType_D_Stat/1  "<FobCtlType_D_Stat>"

== system P702_NI_SoftECU/Output/Subsystem1/CAN_Signal/BCM/Body_Info_4_0x242 ==
  in_port : Inport
  BattULo_I_Actl : Terminator
  BattULo_U_Actl : Terminator
  BrkTrnShifLck_B_Stat : Terminator
  DcacElPw_D_Rq : Terminator
  DriverCrankingReq : Terminator
  EngOff_T_Actl : Terminator
  FuelPumpPwr_D_Stat : Terminator
  PrkLckCtlAvail_T_Stat : Terminator
  PrkLckCtlMsgTxt_D_Rq : Terminator
  PrkLckCtlTow_B_Enbl : Terminator
  PrkLckCtlUnlck_D_Stat : Terminator
  PrkLckCtl_B_Enbl : Terminator
  PtLatchActv_B_RqBcm : Terminator
  ReFuelSwtchStat_D_Actl : Terminator
  bus_selector : BusSelector  OutputSignals=BattULo_I_Actl,BattULo_U_Actl,BrkTrnShifLck_B_Stat,DcacElPw_D_Rq,DriverCrankingReq,EngOff_T_Actl,FuelPumpPwr_D_Stat,PrkLckCtlAvail_T_Stat,PrkLckCtlMsgTxt_D_Rq,PrkLckCtlTow_B_Enbl,PrkLckCtlUnlck_D_Stat,PrkLckCtl_B_Enbl,PtLatchActv_B_RqBcm,ReFuelSwtchStat_D_Actl,immoSecureIdleMode
  immoSecureIdleMode : Terminator
  wires:
  in_port/1 -> bus_selector/1  "Subsystem1"
  bus_selector/1 -> BattULo_I_Actl/1  "<BattULo_I_Actl>"
  bus_selector/2 -> BattULo_U_Actl/1  "<BattULo_U_Actl>"
  bus_selector/3 -> BrkTrnShifLck_B_Stat/1  "<BrkTrnShifLck_B_Stat>"
  bus_selector/4 -> DcacElPw_D_Rq/1  "<DcacElPw_D_Rq>"
  bus_selector/5 -> DriverCrankingReq/1  "<DriverCrankingReq>"
  bus_selector/6 -> EngOff_T_Actl/1  "<EngOff_T_Actl>"
  bus_selector/7 -> FuelPumpPwr_D_Stat/1  "<FuelPumpPwr_D_Stat>"
  bus_selector/8 -> PrkLckCtlAvail_T_Stat/1  "<PrkLckCtlAvail_T_Stat>"
  bus_selector/9 -> PrkLckCtlMsgTxt_D_Rq/1  "<PrkLckCtlMsgTxt_D_Rq>"
  bus_selector/10 -> PrkLckCtlTow_B_Enbl/1  "<PrkLckCtlTow_B_Enbl>"
  bus_selector/11 -> PrkLckCtlUnlck_D_Stat/1  "<PrkLckCtlUnlck_D_Stat>"
  bus_selector/12 -> PrkLckCtl_B_Enbl/1  "<PrkLckCtl_B_Enbl>"
  bus_selector/13 -> PtLatchActv_B_RqBcm/1  "<PtLatchActv_B_RqBcm>"
  bus_selector/14 -> ReFuelSwtchStat_D_Actl/1  "<ReFuelSwtchStat_D_Actl>"
  bus_selector/15 -> immoSecureIdleMode/1  "<immoSecureIdleMode>"

== system P702_NI_SoftECU/Output/Subsystem1/CAN_Signal/BCM/Body_Info_6_0x38D ==
  in_port : Inport
  DrLatchMsgTxt_D_Rq : Terminator
  ElPwPoint_D_Rq : Terminator
  HeadLghtHiPrmsn_D_Stat : Terminator
  IgnPsswrdDsply_B_Rq : Terminator
  KeyAdmnTot_No_Cnt : Terminator
  KeyMykeyTot_No_Cnt : Terminator
  Keycode_Status : Terminator
  PEBackupSlot_Stats : Terminator
  PoliceIdlMde_D_Stat : Terminator
  PrmtrAlrmEvnt_D_Stat : Terminator
  PrsnlDevcChrgEnbl_B_Rq : Terminator
  SecurityMsgTxt_D_Rq : Terminator
  SteWhlLckMsgTxt_D_Rq : Terminator
  TracKeyMde_D_Stat : Terminator
  bus_selector : BusSelector  OutputSignals=KeyAdmnTot_No_Cnt,KeyMykeyTot_No_Cnt,Keycode_Status,PEBackupSlot_Stats,SteWhlLckMsgTxt_D_Rq,immoMsgTxt_D_Rq,PrmtrAlrmEvnt_D_Stat,SecurityMsgTxt_D_Rq,TracKeyMde_D_Stat,DrLatchMsgTxt_D_Rq,PrsnlDevcChrgEnbl_B_Rq,PoliceIdlMde_D_Stat,HeadLghtHiPrmsn_D_Stat,ElPwPoint_D_Rq,IgnPsswrdDsply_B_Rq
  immoMsgTxt_D_Rq : Terminator
  wires:
  in_port/1 -> bus_selector/1  "Subsystem1"
  bus_selector/1 -> KeyAdmnTot_No_Cnt/1  "<KeyAdmnTot_No_Cnt>"
  bus_selector/2 -> KeyMykeyTot_No_Cnt/1  "<KeyMykeyTot_No_Cnt>"
  bus_selector/3 -> Keycode_Status/1  "<Keycode_Status>"
  bus_selector/4 -> PEBackupSlot_Stats/1  "<PEBackupSlot_Stats>"
  bus_selector/5 -> SteWhlLckMsgTxt_D_Rq/1  "<SteWhlLckMsgTxt_D_Rq>"
  bus_selector/6 -> immoMsgTxt_D_Rq/1  "<immoMsgTxt_D_Rq>"
  bus_selector/7 -> PrmtrAlrmEvnt_D_Stat/1  "<PrmtrAlrmEvnt_D_Stat>"
  bus_selector/8 -> SecurityMsgTxt_D_Rq/1  "<SecurityMsgTxt_D_Rq>"
  bus_selector/9 -> TracKeyMde_D_Stat/1  "<TracKeyMde_D_Stat>"
  bus_selector/10 -> DrLatchMsgTxt_D_Rq/1  "<DrLatchMsgTxt_D_Rq>"
  bus_selector/11 -> PrsnlDevcChrgEnbl_B_Rq/1  "<PrsnlDevcChrgEnbl_B_Rq>"
  bus_selector/12 -> PoliceIdlMde_D_Stat/1  "<PoliceIdlMde_D_Stat>"
  bus_selector/13 -> HeadLghtHiPrmsn_D_Stat/1  "<HeadLghtHiPrmsn_D_Stat>"
  bus_selector/14 -> ElPwPoint_D_Rq/1  "<ElPwPoint_D_Rq>"
  bus_selector/15 -> IgnPsswrdDsply_B_Rq/1  "<IgnPsswrdDsply_B_Rq>"

== system P702_NI_SoftECU/Output/Subsystem1/CAN_Signal/BCM/Body_Info_7_0x3B1 ==
  in_port : Inport
  KeyOffMde_D_Actl : Terminator
  bus_selector : BusSelector  OutputSignals=KeyOffMde_D_Actl
  wires:
  in_port/1 -> bus_selector/1  "Subsystem1"
  bus_selector/1 -> KeyOffMde_D_Actl/1  "<KeyOffMde_D_Actl>"

== system P702_NI_SoftECU/Output/Subsystem1/CAN_Signal/BCM/Body_Info_8_0x3B9 ==
  in_port : Inport
  ChrgCordLck_B_Stat : Terminator
  ChrgCordResp1_No_Actl : Terminator
  ChrgCordResp2_No_Actl : Terminator
  WakeAlarm0_D_Stat : Terminator
  WakeAlarm1_D_Stat : Terminator
  WakeAlarm2_D_Stat : Terminator
  WakeAlarm3_D_Stat : Terminator
  bus_selector : BusSelector  OutputSignals=WakeAlarm0_D_Stat,WakeAlarm1_D_Stat,WakeAlarm2_D_Stat,WakeAlarm3_D_Stat,ChrgCordResp1_No_Actl,ChrgCordResp2_No_Actl,ChrgCordLck_B_Stat
  wires:
  in_port/1 -> bus_selector/1  "Subsystem1"
  bus_selector/1 -> WakeAlarm0_D_Stat/1  "<WakeAlarm0_D_Stat>"
  bus_selector/2 -> WakeAlarm1_D_Stat/1  "<WakeAlarm1_D_Stat>"
  bus_selector/3 -> WakeAlarm2_D_Stat/1  "<WakeAlarm2_D_Stat>"
  bus_selector/4 -> WakeAlarm3_D_Stat/1  "<WakeAlarm3_D_Stat>"
  bus_selector/5 -> ChrgCordResp1_No_Actl/1  "<ChrgCordResp1_No_Actl>"
  bus_selector/6 -> ChrgCordResp2_No_Actl/1  "<ChrgCordResp2_No_Actl>"
  bus_selector/7 -> ChrgCordLck_B_Stat/1  "<ChrgCordLck_B_Stat>"

== system P702_NI_SoftECU/Output/Subsystem1/CAN_Signal/BCM/Body_Info_9_0x3A3 ==
  in_port : Inport
  AdvStrt_D_Stat : Terminator
  CrnkInhbt_B_Stat : Terminator
  CrnkInhbt_No_Cnt : Terminator
  CrnkInhbt_No_Cs : Terminator
  DrvInCtl_B_Stat : Terminator
  EngStrtActv_B_Stat : Terminator
  EngStrt_B_Rq : Terminator
  IgnPreOffActv_B_Stat : Terminator
  StrtrMtrCtlDStat_No_Cs : Terminator
  VehOnSrc_D_Stat : Terminator
  bus_selector : BusSelector  OutputSignals=CrnkInhbt_B_Stat,CrnkInhbt_No_Cnt,IgnPreOffActv_B_Stat,DrvInCtl_B_Stat,EngStrt_B_Rq,CrnkInhbt_No_Cs,AdvStrt_D_Stat,VehOnSrc_D_Stat,StrtrMtrCtlDStat_No_Cs,EngStrtActv_B_Stat
  wires:
  in_port/1 -> bus_selector/1  "Subsystem1"
  bus_selector/1 -> CrnkInhbt_B_Stat/1  "<CrnkInhbt_B_Stat>"
  bus_selector/2 -> CrnkInhbt_No_Cnt/1  "<CrnkInhbt_No_Cnt>"
  bus_selector/3 -> IgnPreOffActv_B_Stat/1  "<IgnPreOffActv_B_Stat>"
  bus_selector/4 -> DrvInCtl_B_Stat/1  "<DrvInCtl_B_Stat>"
  bus_selector/5 -> EngStrt_B_Rq/1  "<EngStrt_B_Rq>"
  bus_selector/6 -> CrnkInhbt_No_Cs/1  "<CrnkInhbt_No_Cs>"
  bus_selector/7 -> AdvStrt_D_Stat/1  "<AdvStrt_D_Stat>"
  bus_selector/8 -> VehOnSrc_D_Stat/1  "<VehOnSrc_D_Stat>"
  bus_selector/9 -> StrtrMtrCtlDStat_No_Cs/1  "<StrtrMtrCtlDStat_No_Cs>"
  bus_selector/10 -> EngStrtActv_B_Stat/1  "<EngStrtActv_B_Stat>"

== system P702_NI_SoftECU/Output/Subsystem1/CAN_Signal/BCM/CMPS_FDM_Info_Status_0x3C7 ==
  in_port : Inport
  CamPDCGuidStat : Terminator
  CamZoomActiveState : Terminator
  CamraOvrlDyn_D_Actl : Terminator
  CamraOvrlStat_D_Actl : Terminator
  CamraOvrlTow_D_Actl : Terminator
  CamraViewSplit_D_Actl : Terminator
  CamraZoomMan_D_Actl : Terminator
  bus_selector : BusSelector  OutputSignals=CamraViewSplit_D_Actl,CamraOvrlDyn_D_Actl,CamraZoomMan_D_Actl,CamPDCGuidStat,CamZoomActiveState,CamraOvrlStat_D_Actl,CamraOvrlTow_D_Actl
  wires:
  in_port/1 -> bus_selector/1  "Subsystem1"
  bus_selector/1 -> CamraViewSplit_D_Actl/1  "<CamraViewSplit_D_Actl>"
  bus_selector/2 -> CamraOvrlDyn_D_Actl/1  "<CamraOvrlDyn_D_Actl>"
  bus_selector/3 -> CamraZoomMan_D_Actl/1  "<CamraZoomMan_D_Actl>"
  bus_selector/4 -> CamPDCGuidStat/1  "<CamPDCGuidStat>"
  bus_selector/5 -> CamZoomActiveState/1  "<CamZoomActiveState>"
  bus_selector/6 -> CamraOvrlStat_D_Actl/1  "<CamraOvrlStat_D_Actl>"
  bus_selector/7 -> CamraOvrlTow_D_Actl/1  "<CamraOvrlTow_D_Actl>"

== system P702_NI_SoftECU/Output/Subsystem1/CAN_Signal/BCM/CellPhonePassport_Stat_1_0x447 ==
  in_port : Inport
  HeadLghtOn_D_Rq : Terminator
  KeyProg_No_Actl : Terminator
  PepsKeyActv_D_Stat : Terminator
  PepsKeyFound_No_Actl : Terminator
  Pers1Phone_D_Stat : Terminator
  Pers2Phone_D_Stat : Terminator
  Pers3Phone_D_Stat : Terminator
  Pers4Phone_D_Stat : Terminator
  RstrtSetting_T_Actl : Terminator
  Rstrt_T_Actl : Terminator
  VehLck_D_Dsply : Terminator
  bus_selector : BusSelector  OutputSignals=KeyProg_No_Actl,PepsKeyActv_D_Stat,Rstrt_T_Actl,RstrtSetting_T_Actl,PepsKeyFound_No_Actl,HeadLghtOn_D_Rq,VehLck_D_Dsply,Pers1Phone_D_Stat,Pers2Phone_D_Stat,Pers3Phone_D_Stat,Pers4Phone_D_Stat
  wires:
  in_port/1 -> bus_selector/1  "Subsystem1"
  bus_selector/1 -> KeyProg_No_Actl/1  "<KeyProg_No_Actl>"
  bus_selector/2 -> PepsKeyActv_D_Stat/1  "<PepsKeyActv_D_Stat>"
  bus_selector/3 -> Rstrt_T_Actl/1  "<Rstrt_T_Actl>"
  bus_selector/4 -> RstrtSetting_T_Actl/1  "<RstrtSetting_T_Actl>"
  bus_selector/5 -> PepsKeyFound_No_Actl/1  "<PepsKeyFound_No_Actl>"
  bus_selector/6 -> HeadLghtOn_D_Rq/1  "<HeadLghtOn_D_Rq>"
  bus_selector/7 -> VehLck_D_Dsply/1  "<VehLck_D_Dsply>"
  bus_selector/8 -> Pers1Phone_D_Stat/1  "<Pers1Phone_D_Stat>"
  bus_selector/9 -> Pers2Phone_D_Stat/1  "<Pers2Phone_D_Stat>"
  bus_selector/10 -> Pers3Phone_D_Stat/1  "<Pers3Phone_D_Stat>"
  bus_selector/11 -> Pers4Phone_D_Stat/1  "<Pers4Phone_D_Stat>"

== system P702_NI_SoftECU/Output/Subsystem1/CAN_Signal/BCM/GGCC_Config_Mgmt_ID_1_0x40A ==
  in_port : Inport
  VehicleGGCCData : Terminator
  bus_selector : BusSelector  OutputSignals=VehicleGGCCData
  wires:
  in_port/1 -> bus_selector/1  "Subsystem1"
  bus_selector/1 -> VehicleGGCCData/1  "<VehicleGGCCData>"

== system P702_NI_SoftECU/Output/Subsystem1/CAN_Signal/BCM/GlobalClock_Data_0x84 ==
  in_port : Inport
  GlblClkDay_No_Actl : Terminator
  GlblClkHr_No_Actl : Terminator
  GlblClkMnte_No_Actl : Terminator
  GlblClkScnd_No_Actl : Terminator
  GlblClkYr_No_Actl : Terminator
  bus_selector : BusSelector  OutputSignals=GlblClkYr_No_Actl,GlblClkDay_No_Actl,GlblClkMnte_No_Actl,GlblClkScnd_No_Actl,GlblClkHr_No_Actl
  wires:
  in_port/1 -> bus_selector/1  "Subsystem1"
  bus_selector/1 -> GlblClkYr_No_Actl/1  "<GlblClkYr_No_Actl>"
  bus_selector/2 -> GlblClkDay_No_Actl/1  "<GlblClkDay_No_Actl>"
  bus_selector/3 -> GlblClkMnte_No_Actl/1  "<GlblClkMnte_No_Actl>"
  bus_selector/4 -> GlblClkScnd_No_Actl/1  "<GlblClkScnd_No_Actl>"
  bus_selector/5 -> GlblClkHr_No_Actl/1  "<GlblClkHr_No_Actl>"

== system P702_NI_SoftECU/Output/Subsystem1/CAN_Signal/BCM/Global_PATS_Control_Info2_0x42 ==
  in_port : Inport
  bus_selector : BusSelector  OutputSignals=immoControlCmd_T2,immoControlData_T2
  immoControlCmd_T2 : Terminator
  immoControlData_T2 : Terminator
  wires:
  in_port/1 -> bus_selector/1  "Subsystem1"
  bus_selector/1 -> immoControlCmd_T2/1  "<immoControlCmd_T2>"
  bus_selector/2 -> immoControlData_T2/1  "<immoControlData_T2>"

== system P702_NI_SoftECU/Output/Subsystem1/CAN_Signal/BCM/Global_PATS_Control_Info_0x41 ==
  in_port : Inport
  bus_selector : BusSelector  OutputSignals=immoControlCmd_T1,immoControlData_T1
  immoControlCmd_T1 : Terminator
  immoControlData_T1 : Terminator
  wires:
  in_port/1 -> bus_selector/1  "Subsystem1"
  bus_selector/1 -> immoControlCmd_T1/1  "<immoControlCmd_T1>"
  bus_selector/2 -> immoControlData_T1/1  "<immoControlData_T1>"

== system P702_NI_SoftECU/Output/Subsystem1/CAN_Signal/BCM/Locking_Systems_2_0x331 ==
  in_port : Inport
  ChildLckMde_B_Stat : Terminator
  ChildLck_D_Dsply : Terminator
  DrTgateExtSwMde_B_Stat : Terminator
  DrTgateOpen_B_Rq : Terminator
  FobComm_D_Stat : Terminator
  Keyfob_Pad_Msg_Count : Terminator
  L_Pwr_Sliding_Dr_Rqst : Terminator
  LockInhibit : Terminator
  Lockmsgtxt_D_Rq : Terminator
  Power_Decklid_Rqst : Terminator
  Power_Liftgate_Rqst : Terminator
  R_Pwr_Sliding_Dr_Rqst : Terminator
  Remote_Device_Feedback : Terminator
  RollCodeUnlock : Terminator
  VehLckInd_D_Rq : Terminator
  Veh_Lock_EvNum : Terminator
  Veh_Lock_Requestor : Terminator
  Veh_Lock_Status : Terminator
  Veh_Lock_Sub_Id : Terminator
  WindowLockout_B_Stat : Terminator
  bus_selector : BusSelector  OutputSignals=ChildLck_D_Dsply,FobComm_D_Stat,L_Pwr_Sliding_Dr_Rqst,LockInhibit,Power_Decklid_Rqst,Power_Liftgate_Rqst,Keyfob_Pad_Msg_Count,RollCodeUnlock,Lockmsgtxt_D_Rq,R_Pwr_Sliding_Dr_Rqst,WindowLockout_B_Stat,Veh_Lock_Status,DrTgateExtSwMde_B_Stat,Veh_Lock_EvNum,Veh_Lock_Requestor,Remote_Device_Feedback,Veh_Lock_Sub_Id,DrTgateOpen_B_Rq,VehLckInd_D_Rq,ChildLckMde_B_Stat
  wires:
  in_port/1 -> bus_selector/1  "Subsystem1"
  bus_selector/1 -> ChildLck_D_Dsply/1  "<ChildLck_D_Dsply>"
  bus_selector/2 -> FobComm_D_Stat/1  "<FobComm_D_Stat>"
  bus_selector/3 -> L_Pwr_Sliding_Dr_Rqst/1  "<L_Pwr_Sliding_Dr_Rqst>"
  bus_selector/4 -> LockInhibit/1  "<LockInhibit>"
  bus_selector/5 -> Power_Decklid_Rqst/1  "<Power_Decklid_Rqst>"
  bus_selector/6 -> Power_Liftgate_Rqst/1  "<Power_Liftgate_Rqst>"
  bus_selector/7 -> Keyfob_Pad_Msg_Count/1  "<Keyfob_Pad_Msg_Count>"
  bus_selector/8 -> RollCodeUnlock/1  "<RollCodeUnlock>"
  bus_selector/9 -> Lockmsgtxt_D_Rq/1  "<Lockmsgtxt_D_Rq>"
  bus_selector/10 -> R_Pwr_Sliding_Dr_Rqst/1  "<R_Pwr_Sliding_Dr_Rqst>"
  bus_selector/11 -> WindowLockout_B_Stat/1  "<WindowLockout_B_Stat>"
  bus_selector/12 -> Veh_Lock_Status/1  "<Veh_Lock_Status>"
  bus_selector/13 -> DrTgateExtSwMde_B_Stat/1  "<DrTgateExtSwMde_B_Stat>"
  bus_selector/14 -> Veh_Lock_EvNum/1  "<Veh_Lock_EvNum>"
  bus_selector/15 -> Veh_Lock_Requestor/1  "<Veh_Lock_Requestor>"
  bus_selector/16 -> Remote_Device_Feedback/1  "<Remote_Device_Feedback>"
  bus_selector/17 -> Veh_Lock_Sub_Id/1  "<Veh_Lock_Sub_Id>"
  bus_selector/18 -> DrTgateOpen_B_Rq/1  "<DrTgateOpen_B_Rq>"
  bus_selector/19 -> VehLckInd_D_Rq/1  "<VehLckInd_D_Rq>"
  bus_selector/20 -> ChildLckMde_B_Stat/1  "<ChildLckMde_B_Stat>"

== system P702_NI_SoftECU/Output/Subsystem1/CAN_Signal/BCM/PaakRqData1_0x468 ==
  in_port : Inport
  KeyPadCodeProg_D_Stat : Terminator
  PaakTrgtData_D_Rq : Terminator
  PaakTrgtPssvData_No_Rq : Terminator
  PaakTrgtRollCode_No_Rq : Terminator
  PaakTrgtType_D_Rq : Terminator
  PaakTrgtZone_D_Rq : Terminator
  bus_selector : BusSelector  OutputSignals=PaakTrgtPssvData_No_Rq,PaakTrgtData_D_Rq,PaakTrgtRollCode_No_Rq,PaakTrgtType_D_Rq,PaakTrgtZone_D_Rq,KeyPadCodeProg_D_Stat
  wires:
  in_port/1 -> bus_selector/1  "Subsystem1"
  bus_selector/1 -> PaakTrgtPssvData_No_Rq/1  "<PaakTrgtPssvData_No_Rq>"
  bus_selector/2 -> PaakTrgtData_D_Rq/1  "<PaakTrgtData_D_Rq>"
  bus_selector/3 -> PaakTrgtRollCode_No_Rq/1  "<PaakTrgtRollCode_No_Rq>"
  bus_selector/4 -> PaakTrgtType_D_Rq/1  "<PaakTrgtType_D_Rq>"
  bus_selector/5 -> PaakTrgtZone_D_Rq/1  "<PaakTrgtZone_D_Rq>"
  bus_selector/6 -> KeyPadCodeProg_D_Stat/1  "<KeyPadCodeProg_D_Stat>"

== system P702_NI_SoftECU/Output/Subsystem1/CAN_Signal/BCM/PaakRqData2_0x469 ==
  in_port : Inport
  PaakTrgtActvData_No_Rq : Terminator
  bus_selector : BusSelector  OutputSignals=PaakTrgtActvData_No_Rq
  wires:
  in_port/1 -> bus_selector/1  "Subsystem1"
  bus_selector/1 -> PaakTrgtActvData_No_Rq/1  "<PaakTrgtActvData_No_Rq>"

== system P702_NI_SoftECU/Output/Subsystem1/CAN_Signal/BCM/Personality_BCM2_Data_0x3EB ==
  in_port : Inport
  AssocConfirm_D_Actl : Terminator
  EmPrflKeyAssoc_D_Stat : Terminator
  EmPrflNo_D_Stat : Terminator
  Pers1Key_D_Stat : Terminator
  Pers2Key_D_Stat : Terminator
  Pers3Key_D_Stat : Terminator
  Pers4Key_D_Stat : Terminator
  PersConflict_D_Actl : Terminator
  PersNoPos_D_Actl : Terminator
  PersNo_D_Actl : Terminator
  PersRecallSrc_D_Actl : Terminator
  PersSetupAccessCtrl : Terminator
  PersSetupRestr_D_Actl : Terminator
  PersSetup_No_Actl : Terminator
  RecallEvent_No_Cnt : Terminator
  VehKeyActv_D_Stat : Terminator
  bus_selector : BusSelector  OutputSignals=RecallEvent_No_Cnt,AssocConfirm_D_Actl,Pers1Key_D_Stat,PersNo_D_Actl,PersConflict_D_Actl,PersSetupRestr_D_Actl,PersSetupAccessCtrl,PersNoPos_D_Actl,PersSetup_No_Actl,VehKeyActv_D_Stat,Pers2Key_D_Stat,Pers3Key_D_Stat,EmPrflKeyAssoc_D_Stat,EmPrflNo_D_Stat,Pers4Key_D_Stat,PersRecallSrc_D_Actl
  wires:
  in_port/1 -> bus_selector/1  "Subsystem1"
  bus_selector/1 -> RecallEvent_No_Cnt/1  "<RecallEvent_No_Cnt>"
  bus_selector/2 -> AssocConfirm_D_Actl/1  "<AssocConfirm_D_Actl>"
  bus_selector/3 -> Pers1Key_D_Stat/1  "<Pers1Key_D_Stat>"
  bus_selector/4 -> PersNo_D_Actl/1  "<PersNo_D_Actl>"
  bus_selector/5 -> PersConflict_D_Actl/1  "<PersConflict_D_Actl>"
  bus_selector/6 -> PersSetupRestr_D_Actl/1  "<PersSetupRestr_D_Actl>"
  bus_selector/7 -> PersSetupAccessCtrl/1  "<PersSetupAccessCtrl>"
  bus_selector/8 -> PersNoPos_D_Actl/1  "<PersNoPos_D_Actl>"
  bus_selector/9 -> PersSetup_No_Actl/1  "<PersSetup_No_Actl>"
  bus_selector/10 -> VehKeyActv_D_Stat/1  "<VehKeyActv_D_Stat>"
  bus_selector/11 -> Pers2Key_D_Stat/1  "<Pers2Key_D_Stat>"
  bus_selector/12 -> Pers3Key_D_Stat/1  "<Pers3Key_D_Stat>"
  bus_selector/13 -> EmPrflKeyAssoc_D_Stat/1  "<EmPrflKeyAssoc_D_Stat>"
  bus_selector/14 -> EmPrflNo_D_Stat/1  "<EmPrflNo_D_Stat>"
  bus_selector/15 -> Pers4Key_D_Stat/1  "<Pers4Key_D_Stat>"
  bus_selector/16 -> PersRecallSrc_D_Actl/1  "<PersRecallSrc_D_Actl>"

== system P702_NI_SoftECU/Output/Subsystem1/CAN_Signal/BCM/Personality_BCM_Data_0x3E3 ==
  in_port : Inport
  FeatConfigBcmActl : Terminator
  FeatNoBcm_No_Actl : Terminator
  FobAssocChime_B_Rq : Terminator
  LightAmbColor_No_Actl : Terminator
  LightAmbIntsty_No_Actl : Terminator
  PersIndexBcm_D_Actl : Terminator
  bus_selector : BusSelector  OutputSignals=FeatConfigBcmActl,FeatNoBcm_No_Actl,PersIndexBcm_D_Actl,FobAssocChime_B_Rq,LightAmbColor_No_Actl,LightAmbIntsty_No_Actl
  wires:
  in_port/1 -> bus_selector/1  "Subsystem1"
  bus_selector/1 -> FeatConfigBcmActl/1  "<FeatConfigBcmActl>"
  bus_selector/2 -> FeatNoBcm_No_Actl/1  "<FeatNoBcm_No_Actl>"
  bus_selector/3 -> PersIndexBcm_D_Actl/1  "<PersIndexBcm_D_Actl>"
  bus_selector/4 -> FobAssocChime_B_Rq/1  "<FobAssocChime_B_Rq>"
  bus_selector/5 -> LightAmbColor_No_Actl/1  "<LightAmbColor_No_Actl>"
  bus_selector/6 -> LightAmbIntsty_No_Actl/1  "<LightAmbIntsty_No_Actl>"

== system P702_NI_SoftECU/Output/Subsystem1/CAN_Signal/BCM/Power_Stat_0x456 ==
  in_port : Inport
  RstrnMdulePw_D_Falt : Terminator
  bus_selector : BusSelector  OutputSignals=RstrnMdulePw_D_Falt
  wires:
  in_port/1 -> bus_selector/1  "Subsystem1"
  bus_selector/1 -> RstrnMdulePw_D_Falt/1  "<RstrnMdulePw_D_Falt>"

== system P702_NI_SoftECU/Output/Subsystem1/CAN_Signal/BCM/RKE_Packet_0x3B6 ==
  in_port : Inport
  Modulation_Ctrl : Terminator
  RemoteKey_Info_Ctrl : Terminator
  RemoteKey_Info_Index : Terminator
  RemoteKey_Info_MaxInd : Terminator
  RemoteKey_Info_TIC : Terminator
  TirePress_Filter_Ctrl : Terminator
  bus_selector : BusSelector  OutputSignals=TirePress_Filter_Ctrl,Modulation_Ctrl,RemoteKey_Info_Ctrl,RemoteKey_Info_Index,RemoteKey_Info_MaxInd,RemoteKey_Info_TIC
  wires:
  in_port/1 -> bus_selector/1  "Subsystem1"
  bus_selector/1 -> TirePress_Filter_Ctrl/1  "<TirePress_Filter_Ctrl>"
  bus_selector/2 -> Modulation_Ctrl/1  "<Modulation_Ctrl>"
  bus_selector/3 -> RemoteKey_Info_Ctrl/1  "<RemoteKey_Info_Ctrl>"
  bus_selector/4 -> RemoteKey_Info_Index/1  "<RemoteKey_Info_Index>"
  bus_selector/5 -> RemoteKey_Info_MaxInd/1  "<RemoteKey_Info_MaxInd>"
  bus_selector/6 -> RemoteKey_Info_TIC/1  "<RemoteKey_Info_TIC>"

== system P702_NI_SoftECU/Output/Subsystem1/CAN_Signal/BCM/TPM_Frame_0x3B7 ==
  in_port : Inport
  TirePress_Info_ID : Terminator
  TirePress_Info_Index : Terminator
  TirePress_Info_MaxInd : Terminator
  bus_selector : BusSelector  OutputSignals=TirePress_Info_Index,TirePress_Info_MaxInd,TirePress_Info_ID
  wires:
  in_port/1 -> bus_selector/1  "Subsystem1"
  bus_selector/1 -> TirePress_Info_Index/1  "<TirePress_Info_Index>"
  bus_selector/2 -> TirePress_Info_MaxInd/1  "<TirePress_Info_MaxInd>"
  bus_selector/3 -> TirePress_Info_ID/1  "<TirePress_Info_ID>"

== system P702_NI_SoftECU/Output/Subsystem1/CAN_Signal/BCM/Tire_Pressure_Data_0x3B5 ==
  in_port : Inport
  Tire_Press_LF_Data : Terminator
  Tire_Press_LR_OLR_Data : Terminator
  Tire_Press_RF_Data : Terminator
  Tire_Press_RR_ORR_Data : Terminator
  bus_selector : BusSelector  OutputSignals=Tire_Press_LF_Data,Tire_Press_RF_Data,Tire_Press_RR_ORR_Data,Tire_Press_LR_OLR_Data
  wires:
  in_port/1 -> bus_selector/1  "Subsystem1"
  bus_selector/1 -> Tire_Press_LF_Data/1  "<Tire_Press_LF_Data>"
  bus_selector/2 -> Tire_Press_RF_Data/1  "<Tire_Press_RF_Data>"
  bus_selector/3 -> Tire_Press_RR_ORR_Data/1  "<Tire_Press_RR_ORR_Data>"
  bus_selector/4 -> Tire_Press_LR_OLR_Data/1  "<Tire_Press_LR_OLR_Data>"

== system P702_NI_SoftECU/Output/Subsystem1/CAN_Signal/BCM/Tire_Pressure_Data_DRW_0x3B8 ==
  in_port : Inport
  Tire_Press_ILR_Data : Terminator
  Tire_Press_IRR_Data : Terminator
  bus_selector : BusSelector  OutputSignals=Tire_Press_ILR_Data,Tire_Press_IRR_Data
  wires:
  in_port/1 -> bus_selector/1  "Subsystem1"
  bus_selector/1 -> Tire_Press_ILR_Data/1  "<Tire_Press_ILR_Data>"
  bus_selector/2 -> Tire_Press_IRR_Data/1  "<Tire_Press_IRR_Data>"

== system P702_NI_SoftECU/Output/Subsystem1/CAN_Signal/BCM/Tire_Pressure_Stat_0x3B4 ==
  in_port : Inport
  TirePReset_D_Stat : Terminator
  Tire_Press_ILR_Stat : Terminator
  Tire_Press_IRR_Stat : Terminator
  Tire_Press_LF_Stat : Terminator
  Tire_Press_LR_OLR_Stat : Terminator
  Tire_Press_Placrd_Frnt : Terminator
  Tire_Press_Placrd_Rear : Terminator
  Tire_Press_RF_Stat : Terminator
  Tire_Press_RR_ORR_Stat : Terminator
  Tire_Press_System_Stat : Terminator
  Tire_Press_Telltale : Terminator
  bus_selector : BusSelector  OutputSignals=Tire_Press_System_Stat,Tire_Press_Telltale,TirePReset_D_Stat,Tire_Press_LF_Stat,Tire_Press_RF_Stat,Tire_Press_RR_ORR_Stat,Tire_Press_LR_OLR_Stat,Tire_Press_IRR_Stat,Tire_Press_ILR_Stat,Tire_Press_Placrd_Frnt,Tire_Press_Placrd_Rear
  wires:
  in_port/1 -> bus_selector/1  "Subsystem1"
  bus_selector/1 -> Tire_Press_System_Stat/1  "<Tire_Press_System_Stat>"
  bus_selector/2 -> Tire_Press_Telltale/1  "<Tire_Press_Telltale>"
  bus_selector/3 -> TirePReset_D_Stat/1  "<TirePReset_D_Stat>"
  bus_selector/4 -> Tire_Press_LF_Stat/1  "<Tire_Press_LF_Stat>"
  bus_selector/5 -> Tire_Press_RF_Stat/1  "<Tire_Press_RF_Stat>"
  bus_selector/6 -> Tire_Press_RR_ORR_Stat/1  "<Tire_Press_RR_ORR_Stat>"
  bus_selector/7 -> Tire_Press_LR_OLR_Stat/1  "<Tire_Press_LR_OLR_Stat>"
  bus_selector/8 -> Tire_Press_IRR_Stat/1  "<Tire_Press_IRR_Stat>"
  bus_selector/9 -> Tire_Press_ILR_Stat/1  "<Tire_Press_ILR_Stat>"
  bus_selector/10 -> Tire_Press_Placrd_Frnt/1  "<Tire_Press_Placrd_Frnt>"
  bus_selector/11 -> Tire_Press_Placrd_Rear/1  "<Tire_Press_Placrd_Rear>"

== system P702_NI_SoftECU/Output/Subsystem1/CAN_Signal/DSMC/CMR_DSMC_AutoSar_NetwrkMgt ==
  in_port : Inport
  CMR_DSMC_AutoSarNMControl : Terminator
  CMR_DSMC_AutoSarNMNodeId : Terminator
  CMR_DSMC_AutoSarNMReserve2 : Terminator
  CMR_DSMC_AutoSarNMReserve3 : Terminator
  CMR_DSMC_AutoSarNMReserve4 : Terminator
  CMR_DSMC_AutoSarNMReserved : Terminator
  CMR_DSMC_GWNMProxY : Terminator
  CMR_DSMC_GWOnBoardTester : Terminator
  bus_selector : BusSelector  OutputSignals=CMR_DSMC_AutoSarNMControl,CMR_DSMC_AutoSarNMNodeId,CMR_DSMC_AutoSarNMReserve2,CMR_DSMC_AutoSarNMReserve3,CMR_DSMC_AutoSarNMReserve4,CMR_DSMC_AutoSarNMReserved,CMR_DSMC_GWNMProxY,CMR_DSMC_GWOnBoardTester
  wires:
  in_port/1 -> bus_selector/1  "Subsystem1"
  bus_selector/1 -> CMR_DSMC_AutoSarNMControl/1  "<CMR_DSMC_AutoSarNMControl>"
  bus_selector/2 -> CMR_DSMC_AutoSarNMNodeId/1  "<CMR_DSMC_AutoSarNMNodeId>"
  bus_selector/3 -> CMR_DSMC_AutoSarNMReserve2/1  "<CMR_DSMC_AutoSarNMReserve2>"
  bus_selector/4 -> CMR_DSMC_AutoSarNMReserve3/1  "<CMR_DSMC_AutoSarNMReserve3>"
  bus_selector/5 -> CMR_DSMC_AutoSarNMReserve4/1  "<CMR_DSMC_AutoSarNMReserve4>"
  bus_selector/6 -> CMR_DSMC_AutoSarNMReserved/1  "<CMR_DSMC_AutoSarNMReserved>"
  bus_selector/7 -> CMR_DSMC_GWNMProxY/1  "<CMR_DSMC_GWNMProxY>"
  bus_selector/8 -> CMR_DSMC_GWOnBoardTester/1  "<CMR_DSMC_GWOnBoardTester>"

== system P702_NI_SoftECU/Output/Subsystem1/CAN_Signal/DSMC/DrvStatMonData ==
  in_port : Inport
  DrvAlertSt_D_Stat : Terminator
  DrvAttentZone_D_Stat : Terminator
  DrvCamDrvIR_D_Stat : Terminator
  DrvCamPassIR_D_Stat : Terminator
  DrvCamera_D_Stat : Terminator
  DrvEngLvlConfid_D_Stat : Terminator
  DrvEngageLevel_D_Stat : Terminator
  DrvEngageLevel_No_Cnt : Terminator
  DrvEngageLevel_No_Cs : Terminator
  DrvImpLvlConfid_D_Stat : Terminator
  DrvImpairLvl_D_Stat : Terminator
  bus_selector : BusSelector  OutputSignals=DrvAlertSt_D_Stat,DrvAttentZone_D_Stat,DrvCamDrvIR_D_Stat,DrvCamPassIR_D_Stat,DrvCamera_D_Stat,DrvEngLvlConfid_D_Stat,DrvEngageLevel_D_Stat,DrvEngageLevel_No_Cnt,DrvEngageLevel_No_Cs,DrvImpLvlConfid_D_Stat,DrvImpairLvl_D_Stat
  wires:
  in_port/1 -> bus_selector/1  "Subsystem1"
  bus_selector/1 -> DrvAlertSt_D_Stat/1  "<DrvAlertSt_D_Stat>"
  bus_selector/2 -> DrvAttentZone_D_Stat/1  "<DrvAttentZone_D_Stat>"
  bus_selector/3 -> DrvCamDrvIR_D_Stat/1  "<DrvCamDrvIR_D_Stat>"
  bus_selector/4 -> DrvCamPassIR_D_Stat/1  "<DrvCamPassIR_D_Stat>"
  bus_selector/5 -> DrvCamera_D_Stat/1  "<DrvCamera_D_Stat>"
  bus_selector/6 -> DrvEngLvlConfid_D_Stat/1  "<DrvEngLvlConfid_D_Stat>"
  bus_selector/7 -> DrvEngageLevel_D_Stat/1  "<DrvEngageLevel_D_Stat>"
  bus_selector/8 -> DrvEngageLevel_No_Cnt/1  "<DrvEngageLevel_No_Cnt>"
  bus_selector/9 -> DrvEngageLevel_No_Cs/1  "<DrvEngageLevel_No_Cs>"
  bus_selector/10 -> DrvImpLvlConfid_D_Stat/1  "<DrvImpLvlConfid_D_Stat>"
  bus_selector/11 -> DrvImpairLvl_D_Stat/1  "<DrvImpairLvl_D_Stat>"

== system P702_NI_SoftECU/Output/Subsystem1/CAN_Signal/DSMC/TesterPhysicalResCMR_DSMC ==
  in_port : Inport
  TesterPhysicalResCMR_DSMC : Terminator
  bus_selector : BusSelector  OutputSignals=TesterPhysicalResCMR_DSMC
  wires:
  in_port/1 -> bus_selector/1  "Subsystem1"
  bus_selector/1 -> TesterPhysicalResCMR_DSMC/1  "<TesterPhysicalResCMR_DSMC>"
